simulink model "A01_Heater1_Random"  (R2016a)
settings: Solver=ode45  StartTime=0.0  StopTime=7700  RelTol=1e-3
StartFcn:
  | clear all
libraries: realtime_pacer_lib x1
settings Model: Creator=johnh  LastModifiedBy=tiago
settings DataIOCC: SaveFormat=StructureWithTime
settings OptimizationCC: BlockReduction=off  DefaultParameterBehavior=Inlined  BufferReuse=off
settings HardwareCC: ProdWordSize=32  ProdHWDeviceType=Specified
settings ConfigComp: CovModelRefEnable=Off

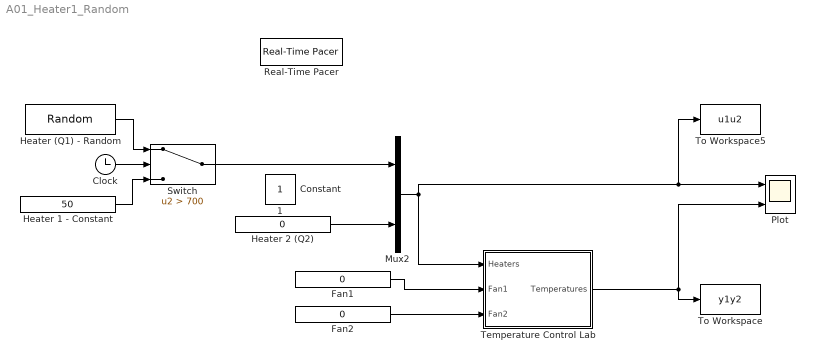
== system A01_Heater1_Random ==
  Clock : Clock
  Fan1 : Constant  Value=0
  Fan2 : Constant  Value=0
  Heater (Q1) - Random : RandomNumber  Mean=50  Variance=200  Seed=4  SampleTime=35
  Heater 1 - Constant : Constant  Value=50
  Heater 2 (Q2) : Constant  Value=0
  Mux2 : Mux  Inputs=2
  Plot : Scope  NumInputPorts=2
  Real-Time Pacer : realtime_pacer_lib/Real-Time Pacer  simTimePerRealTime=1
  Switch : Switch  Criteria=u2 > Threshold  Threshold=700
  Temperature Control Lab : Subsystem
      mask Display: image('tclab.png');
  To Workspace : ToWorkspace  VariableName=y1y2  SaveFormat=Timeseries  SampleTime=-1
  To Workspace5 : ToWorkspace  VariableName=u1u2  SaveFormat=Timeseries  SampleTime=-1
  1 : Constant  IOType=siggen
  Constant : Constant  IOType=siggen
  wires:
  Heater 2 (Q2)/1 -> Mux2/2
  Temperature Control Lab/1(Temperatures) -> Plot/2, To Workspace/1
  Mux2/1 -> Temperature Control Lab/1(Heaters), To Workspace5/1, Plot/1
  Clock/1 -> Switch/2
  Switch/1 -> Mux2/1
  Heater (Q1) - Random/1 -> Switch/1
  Heater 1 - Constant/1 -> Switch/3
  Fan2/1 -> Temperature Control Lab/3(Fan2)
  Fan1/1 -> Temperature Control Lab/2(Fan1)

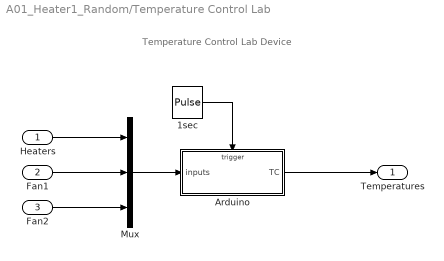
== system A01_Heater1_Random/Temperature Control Lab ==
  note: Temperature Control Lab Device
  Heaters : Inport  PortDimensions=2
  Fan1 : Inport  Port=2  PortDimensions=1
  Fan2 : Inport  Port=3  PortDimensions=1
  1sec : DiscretePulseGenerator  PulseType=Time based  Period=0.5  PulseWidth=50
  Arduino : Subsystem  TreatAsAtomicUnit=on
  Mux : Mux  Inputs=3
  Temperatures : Outport
  wires:
  1sec/1 -> Arduino/Trigger
  Arduino/1(TC) -> Temperatures/1
  Mux/1 -> Arduino/1(inputs)
  Heaters/1 -> Mux/1
  Fan2/1 -> Mux/3
  Fan1/1 -> Mux/2

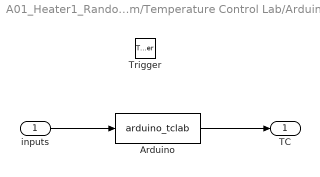
== system A01_Heater1_Random/Temperature Control Lab/Arduino ==
  inputs : Inport  PortDimensions=4  LatchByDelayingOutsideSignal=on
  Trigger : TriggerPort  VariantControl=Variant
  Arduino : MATLABFcn  MATLABFcn=arduino_tclab
  TC : Outport  InitialOutput=[23 23]
  wires:
  inputs/1 -> Arduino/1
  Arduino/1 -> TC/1
